simulink model "wander2"  (R2021b)
settings: Solver=ode3  StartTime=0.0  StopTime=inf  FixedStep=0.05  RelTol=1e-3  EnableMultiTasking=on
undefined symbols (not defined in the file): Angular, Linear
libraries: robotlib x3
settings Model: Creator=The MathWorks, Inc.  LastModifiedBy=vasud
settings SolverCC: AlgebraicLoopSolver=TrustRegion
settings DataIOCC: ReturnWorkspaceOutputs=off
settings OptimizationCC: EnhancedBackFolding=on  PassReuseOutputArgsAs=Individual arguments  ZeroExternalMemoryAtStartup=off  ZeroInternalMemoryAtStartup=off  MaxStackSize=64  OptimizeBlockOrder=speed  DifferentSizesBufferReuse=on  OptimizationCustomize=off  EfficientTunableParamExpr=on
settings DebuggingCC: ParameterTunabilityLossMsg=error  SFMachineParentedDataDiag=warning  ArithmeticOperatorsInVariantConditions=warning
settings HardwareCC: ProdBitPerPointer=32  ProdBitPerSizeT=32  ProdBitPerPtrDiffT=32  ProdLargestAtomicFloat=None  ProdIntDivRoundTo=Undefined  ProdEndianess=Unspecified  ProdWordSize=32  ProdHWDeviceType=Generic->Unspecified (assume 32-bit Generic)
settings SFSimCC: SimUseLocalCustomCode=off  MATLABDynamicMemAlloc=off  CustomCodeUndefinedFunction=UseInterfaceOnly
settings RTWCC: Description=Embedded Coder  SystemTargetFile=ert.tlc  HardwareBoard=Robot Operating System (ROS)  TLCOptions="-aInlineSetEventsForThisBaseRateFcn=TLC_FALSE -aSuppressMultiTaskScheduler=TLC_FALSE  -aRateBasedStepFcn=0"  TemplateMakefile=ert_default_tmf  RTWUseLocalCustomCode=off  Toolchain=Catkin  TargetLang=C++
settings CodeAppCC: ForceParamTrailComments=on  IgnoreCustomStorageClasses=off  OperatorAnnotations=on  SimulinkDataObjDesc=on  SFDataObjDesc=on  InsertBlockDesc=on
settings ERTTargetCC: SupportVariableSizeSignals=on
settings ConfigComp: CovMetricSettings=dsw  CovSaveCumulativeToWorkspaceVar=on  CovSaveSingleToWorkspaceVar=on  CovExternalEMLEnable=off

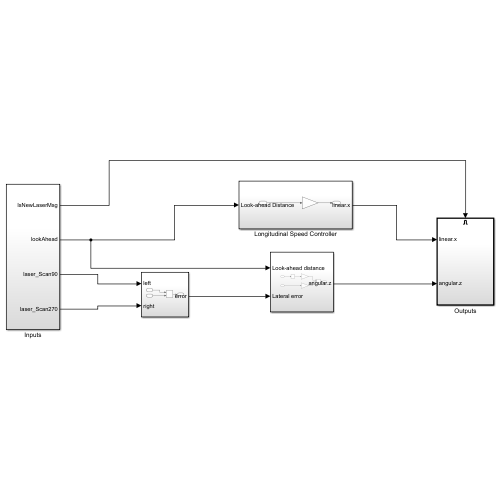
[thumbnail: Simulink's stored preview of the top-level diagram]
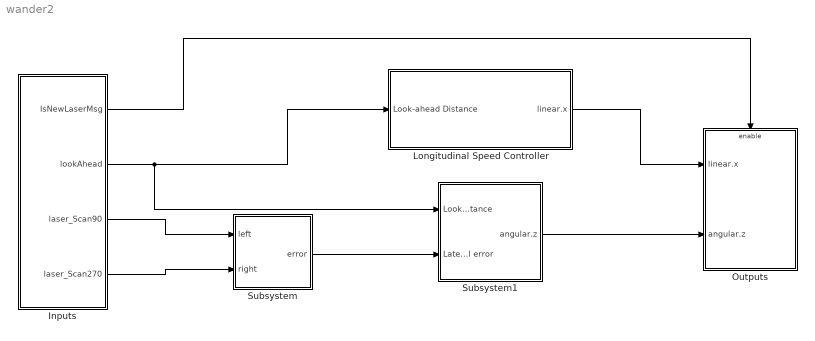
== system wander2 ==
  Inputs : Subsystem
  Longitudinal Speed Controller : Subsystem
  Outputs : Subsystem
  Subsystem : Subsystem
  Subsystem1 : Subsystem
  wires:
  Inputs/1(IsNewLaserMsg) -> Outputs/Enable
  Inputs/3(laser_Scan90) -> Subsystem/1(left)
  Inputs/4(laser_Scan270) -> Subsystem/2(right)
  Subsystem/1(error) -> Subsystem1/2(Lateral error)
  Inputs/2(lookAhead) -> Subsystem1/1(Look-ahead distance), Longitudinal Speed Controller/1(Look-ahead Distance)
  Longitudinal Speed Controller/1(linear.x) -> Outputs/1(linear.x)
  Subsystem1/1(angular.z) -> Outputs/2(angular.z)

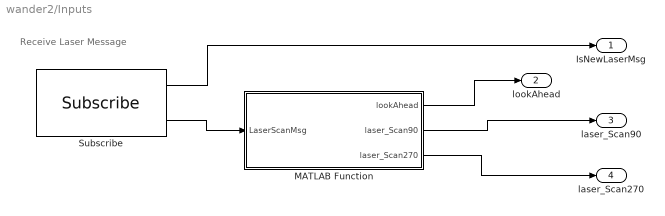
== system wander2/Inputs ==
  note: Receive Laser Message
  MATLAB Function : MATLAB Function  TreatAsAtomicUnit=on
  Subscribe : robotlib/Subscribe  topicSource=Select from ROS network  topic=/scan  messageType=sensor_msgs/LaserScan  SampleTime=-1  legacyBusStruct=off  messageQueueLength=1
  IsNewLaserMsg : Outport  VectorParamsAs1DForOutWhenUnconnected=off
  lookAhead : Outport  Port=2  VectorParamsAs1DForOutWhenUnconnected=off
  laser_Scan90 : Outport  Port=3  VectorParamsAs1DForOutWhenUnconnected=off
  laser_Scan270 : Outport  Port=4  VectorParamsAs1DForOutWhenUnconnected=off
  wires:
  Subscribe/2 -> MATLAB Function/1(LaserScanMsg)
  MATLAB Function/1(lookAhead) -> lookAhead/1
  MATLAB Function/2(laser_Scan90) -> laser_Scan90/1
  Subscribe/1 -> IsNewLaserMsg/1
  MATLAB Function/3(laser_Scan270) -> laser_Scan270/1

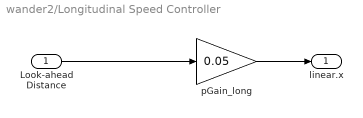
== system wander2/Longitudinal Speed Controller ==
  Look-ahead Distance : Inport
  pGain_long : Gain  Gain=0.05  OutDataTypeStr=single
  linear.x : Outport
  wires:
  Look-ahead Distance/1 -> pGain_long/1
  pGain_long/1 -> linear.x/1

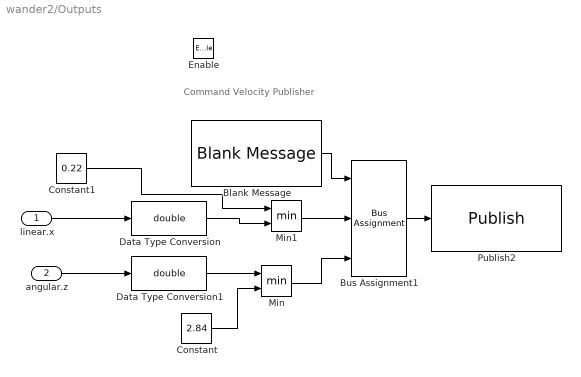
== system wander2/Outputs ==
  note: Command Velocity Publisher
  linear.x : Inport
  angular.z : Inport  Port=2
  Enable : EnablePort
  Blank Message : robotlib/Blank Message  messageClass=Message  entityType=geometry_msgs/Twist  messageType=geometry_msgs/Twist  SampleTime=inf  legacyBusStruct=off
  Bus Assignment1 : BusAssignment  DialogController=Simulink.DDGSource_BusAssignment  AssignedSignals=Linear.X,Angular.Z
  Constant : Constant  Value=2.84
  Constant1 : Constant  Value=0.22
  Data Type Conversion : DataTypeConversion  OutDataTypeStr=double
  Data Type Conversion1 : DataTypeConversion  OutDataTypeStr=double
  Min : MinMax  Inputs=2
  Min1 : MinMax  Inputs=2
  Publish2 : robotlib/Publish  topicSource=Specify your own  topic=/cmd_vel  messageType=geometry_msgs/Twist  legacyBusStruct=off  messageQueueLength=105
  wires:
  angular.z/1 -> Data Type Conversion1/1
  linear.x/1 -> Data Type Conversion/1
  Blank Message/1 -> Bus Assignment1/1
  Bus Assignment1/1 -> Publish2/1
  Constant/1 -> Min/2
  Data Type Conversion1/1 -> Min/1
  Min/1 -> Bus Assignment1/3
  Min1/1 -> Bus Assignment1/2
  Data Type Conversion/1 -> Min1/2
  Constant1/1 -> Min1/1

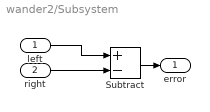
== system wander2/Subsystem ==
  left : Inport
  right : Inport  Port=2
  Subtract : Sum  Inputs=+-
  error : Outport
  wires:
  Subtract/1 -> error/1
  right/1 -> Subtract/2
  left/1 -> Subtract/1

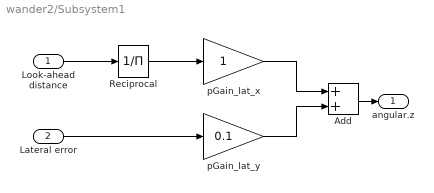
== system wander2/Subsystem1 ==
  Look-ahead distance : Inport
  Lateral error : Inport  Port=2
  Add : Sum
  Reciprocal : Product  Inputs=/
  pGain_lat_x : Gain  OutDataTypeStr=single
  pGain_lat_y : Gain  Gain=0.1  OutDataTypeStr=single
  angular.z : Outport
  wires:
  pGain_lat_y/1 -> Add/2
  Lateral error/1 -> pGain_lat_y/1
  Add/1 -> angular.z/1
  pGain_lat_x/1 -> Add/1
  Reciprocal/1 -> pGain_lat_x/1
  Look-ahead distance/1 -> Reciprocal/1

== matlab function wander2/Inputs/MATLAB Function ==
  data: LaserScanMsg input; lookAhead output; laser_Scan90 output; laser_Scan270 output
function [lookAhead, laser_Scan90, laser_Scan270] = ExtractRangeData(LaserScanMsg)
%#codegen

% Extract Range information
window = 5;
lookAhead = min(3.5,(sum(LaserScanMsg.Ranges(1:10)+LaserScanMsg.Ranges(351:360))/20));
laser_Scan90 = min(3.5,(sum(LaserScanMsg.Ranges(90-window:90+window)/20)));
laser_Scan270 = min(3.5,(sum(LaserScanMsg.Ranges(269-window:269+window)/(2*window))));
